simulink model "intelligent_improved_acceleration_function"  (R2024b)
settings: Solver=VariableStepAuto  StartTime=0.0  StopTime=80  RelTol=1e-3
libraries: SignalEditorBlockLib x6
settings Model: Creator=ky  LastModifiedBy=ky

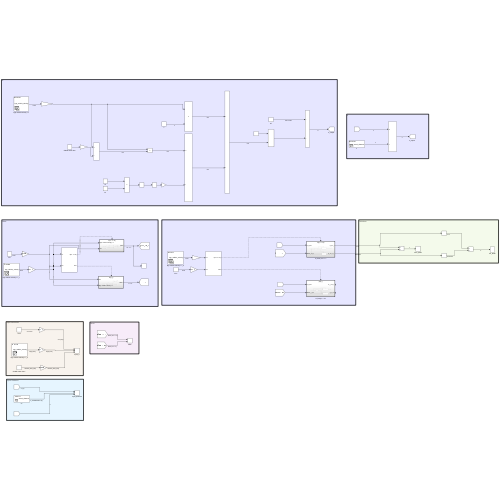
[thumbnail: Simulink's stored preview of the top-level diagram]
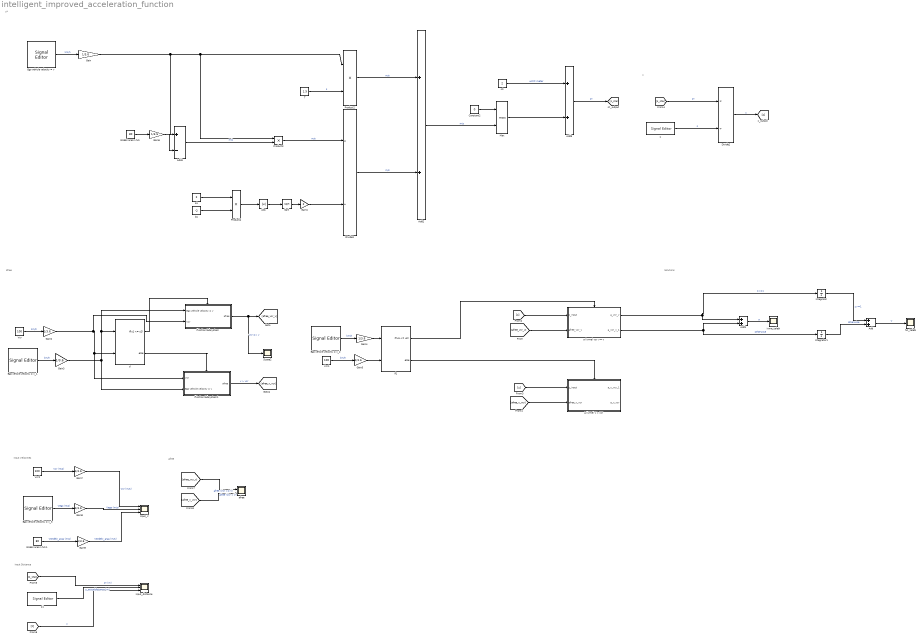
== system intelligent_improved_acceleration_function ==
  note: afree
  note: Solutions
  note: Input Distance
  note: Input Velocities
  note: s*
  note: z
  note: afree
  Abs : Abs  SaturateOnIntegerOverflow=off
  Add{,1..3} (4 alike) : Sum
  Add4 : Sum  Inputs=+-
  Constant2 : Constant  Value=0
  Divide2 : Product  Inputs=*/
  Divide3 : Product  Inputs=*/
  Ego vehicle velocity = v : SignalEditorBlockLib/Signal Editor  FileName=C:\Users\ky\Desktop\MATLAB\otonom_surus\ego_vehicle_velocity.mat  ActiveScenario=Scenario  ActiveSignal=ego_vehicle_velocity  IsBus=off  OutputBusObjectStr=Bus: BusObject  SampleTime=0  ZeroCross=off  OutputAfterFinalValue=Setting to zero  Unit=km/h  PreserveSignalName=on  ApplySigPropsToAllScenarios=on  ApplySigPropsToAllSignals=off
  Ego vehicle velocity = v_1 : SignalEditorBlockLib/Signal Editor  FileName=C:\Users\ky\Desktop\MATLAB\otonom_surus\ego_vehicle_velocity.mat  ActiveScenario=Scenario  ActiveSignal=ego_vehicle_velocity  IsBus=off  OutputBusObjectStr=Bus: BusObject  SampleTime=0  ZeroCross=off  OutputAfterFinalValue=Setting to zero  Unit=km/h  PreserveSignalName=on  ApplySigPropsToAllScenarios=on  ApplySigPropsToAllSignals=off
  Ego vehicle velocity = v_2 : SignalEditorBlockLib/Signal Editor  FileName=C:\Users\ky\Desktop\MATLAB\otonom_surus\ego_vehicle_velocity.mat  ActiveScenario=Scenario  ActiveSignal=ego_vehicle_velocity  IsBus=off  OutputBusObjectStr=Bus: BusObject  SampleTime=0  ZeroCross=off  OutputAfterFinalValue=Setting to zero  Unit=km/h  PreserveSignalName=on  ApplySigPropsToAllScenarios=on  ApplySigPropsToAllSignals=off
  Ego vehicle velocity = v_3 : SignalEditorBlockLib/Signal Editor  FileName=C:\Users\ky\Desktop\MATLAB\otonom_surus\ego_vehicle_velocity.mat  ActiveScenario=Scenario  ActiveSignal=ego_vehicle_velocity  IsBus=off  OutputBusObjectStr=Bus: BusObject  SampleTime=0  ZeroCross=off  OutputAfterFinalValue=Setting to zero  Unit=km/h  PreserveSignalName=on  ApplySigPropsToAllScenarios=on  ApplySigPropsToAllSignals=off
  Gain{,2..9} (9 alike) : Gain  Gain=1/3.6
  Gain1 : Gain  Gain=2
  If : If  NumInputs=2  IfExpression=u1 <= u2
  If Action Subsystem : Subsystem  TreatAsAtomicUnit=on
  If Action Subsystem1 : Subsystem  TreatAsAtomicUnit=on
  If1 : If  NumInputs=2  IfExpression=u1 <= u2
  Input_V : Scope  NumInputPorts=3
  Input_distance : Scope  NumInputPorts=3
  Integrator : Integrator
  Integrator1 : Integrator
  Max : MinMax  Function=max  Inputs=2
  Product2 : Product
  Product3 : Product
  Product4 : Product
  Scope2 : Scope
  Sqrt : Sqrt
  T : Constant  Value=1.5
  Vcr : Constant  Value=100
  Vcr1 : Constant  Value=100
  Vcr2 : Constant  Value=100
  a (ivme) v > vcr : Subsystem  TreatAsAtomicUnit=on
  a (ivme) vcr >= v : Subsystem  TreatAsAtomicUnit=on
  a1 : Constant  Value=2
  afree : Scope  NumInputPorts=2
  b1 : Constant  Value=-2
  hız_talebi : Scope
  ivme_talebi : Scope
  s : SignalEditorBlockLib/Signal Editor  FileName=C:\Users\ky\Desktop\MATLAB\otonom_surus\actual_distance.mat  ActiveScenario=Scenario  ActiveSignal=actual_distance  IsBus=off  OutputBusObjectStr=Bus: BusObject  SampleTime=0  ZeroCross=off  OutputAfterFinalValue=Setting to zero  Unit=m  PreserveSignalName=on  ApplySigPropsToAllScenarios=on  ApplySigPropsToAllSignals=off
  s0 : Constant  Value=2
  s1 : SignalEditorBlockLib/Signal Editor  FileName=C:\Users\ky\Desktop\MATLAB\otonom_surus\actual_distance.mat  ActiveScenario=Scenario  ActiveSignal=actual_distance  IsBus=off  OutputBusObjectStr=Bus: BusObject  SampleTime=0  ZeroCross=off  OutputAfterFinalValue=Setting to zero  Unit=m  PreserveSignalName=on  ApplySigPropsToAllScenarios=on  ApplySigPropsToAllSignals=off
  öndeki aracın hızı : Constant  Value=80
  öndeki aracın hızı1 : Constant  Value=80
  wires:
  Vcr/1 -> Gain2/1  "km/h"
  s1/1 -> Input_distance/2  "s_actualdistance (m)"
  Add4/1 -> Product3/2  "m/s"
  Divide2/1 -> [z]  "z"
  Product3/1 -> Divide3/1  "m/s"
  öndeki aracın hızı1/1 -> Gain9/1  "Vöndeki_araç (m/s)"
  a (ivme) vcr >= v/2(a_vcr_v_1) -> Add1/2, Integrator1/1  "otherwise"
  Product2/1 -> Add2/1  "m/s"
  Ego vehicle velocity = v_1/1 -> Gain3/1  "km/h"
  öndeki aracın hızı/1 -> Gain6/1
  Gain3/1 -> If Action Subsystem1/2(Ego vehicle velocity = v), If Action Subsystem/1(Ego vehicle velocity = v), If/1
  Gain8/1 -> Input_V/2  "Vego (m/s)"
  Add3/1 -> [s_star]  "s*"
  Vcr2/1 -> Gain7/1  "Vcr (m/s)"
  Gain5/1 -> If1/2
  If Action Subsystem1/1(afree) -> [afree_v_vcr]  "v > vcr"
  Abs/1 -> Sqrt/1
  If Action Subsystem/1(afree) -> Scope2/1, [afree_vcr_v]  "vcr => v"
  a (ivme) vcr >= v/1(a_vcr_v) -> Integrator/1, Add1/1  "z>=1"
  Gain4/1 -> If1/1
  [afree_v_vcr] -> a (ivme) v > vcr/2(afree_v_vcr)
  b1/1 -> Product4/2
  Ego vehicle velocity = v_3/1 -> Gain8/1  "Vego (m/s)"
  T/1 -> Product2/2  "s"
  [s_star] -> Divide2/1  "s*"
  Gain/1 -> Add4/1, Product2/1, Product3/1
  Divide3/1 -> Add2/2  "m/s"
  Add2/1 -> Max/2  "m/s"
  s0/1 -> Add3/1  "unit= meter"
  [afree_vcr_v] -> a (ivme) vcr >= v/2(afree_vcr_v)
  If/2 -> If Action Subsystem1/Action
  Gain9/1 -> Input_V/3  "Vöndeki_araç (m/s)"
  [z] -> a (ivme) vcr >= v/1(z_input)
  Constant2/1 -> Max/1
  [z] -> a (ivme) v > vcr/1(z_input)
  Ego vehicle velocity = v/1 -> Gain/1  "km/h"
  Gain7/1 -> Input_V/1  "Vcr (m/s)"
  [s_star] -> Input_distance/1  "s* (m)"
  Sqrt/1 -> Gain1/1
  Gain2/1 -> If Action Subsystem/2(Vcr), If Action Subsystem1/1(Vcr), If/2
  Product4/1 -> Abs/1
  Max/1 -> Add3/2
  Ego vehicle velocity = v_2/1 -> Gain4/1  "km/h"
  s/1 -> Divide2/2  "s"
  If1/1 -> a (ivme) vcr >= v/Action
  [z] -> Input_distance/3  "z"
  If1/2 -> a (ivme) v > vcr/Action
  a1/1 -> Product4/1
  Vcr1/1 -> Gain5/1  "km/h"
  Integrator/1 -> Add/1  "z>=1"
  Gain1/1 -> Divide3/2
  Add1/1 -> ivme_talebi/1  "a"
  Gain6/1 -> Add4/2
  If/1 -> If Action Subsystem/Action
  Add/1 -> hız_talebi/1  "V"
  Integrator1/1 -> Add/2  "otherwise"
  [afree_vcr_v] -> afree/1  "afree (Vcr >= V)"
  [afree_v_vcr] -> afree/2  "afree (Vcr < V)"

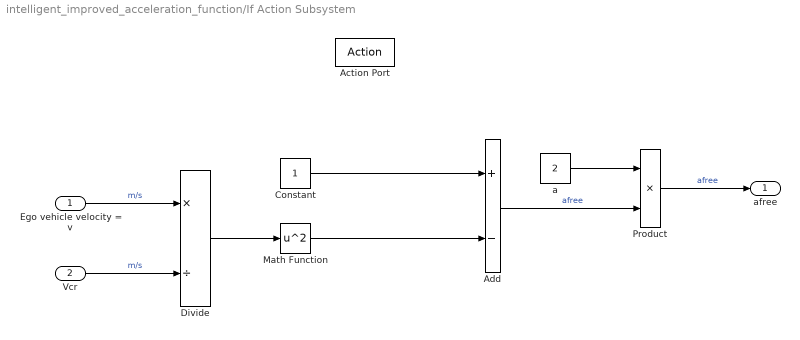
== system intelligent_improved_acceleration_function/If Action Subsystem ==
  Ego vehicle velocity = v : Inport
  Vcr : Inport  Port=2
  Action Port : ActionPort  ActionPortLabel=if(u1 <= u2)
  Add : Sum  Inputs=+-
  Constant : Constant
  Divide : Product  Inputs=*/
  Math Function : Math  Operator=square
  Product : Product
  a : Constant  Value=2
  afree : Outport
  wires:
  Constant/1 -> Add/1
  Math Function/1 -> Add/2
  Divide/1 -> Math Function/1
  a/1 -> Product/1
  Vcr/1 -> Divide/2  "m/s"
  Product/1 -> afree/1  "afree"
  Add/1 -> Product/2  "afree"
  Ego vehicle velocity = v/1 -> Divide/1  "m/s"

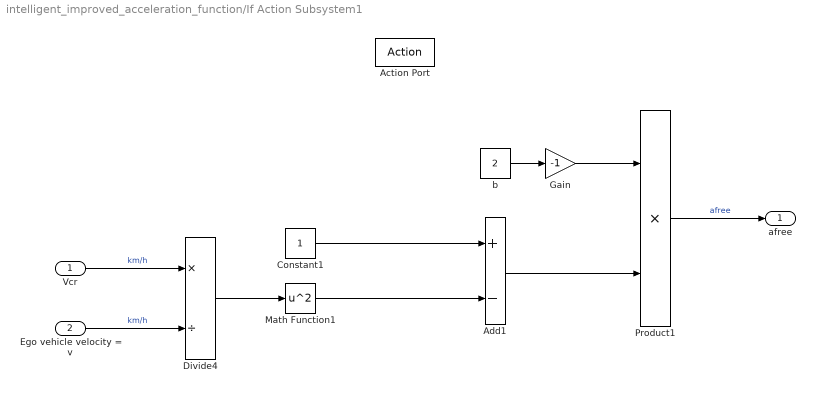
== system intelligent_improved_acceleration_function/If Action Subsystem1 ==
  Vcr : Inport
  Ego vehicle velocity = v : Inport  Port=2
  Action Port : ActionPort  ActionPortLabel=else
  Add1 : Sum  Inputs=+-
  Constant1 : Constant
  Divide4 : Product  Inputs=*/
  Gain : Gain  Gain=-1
  Math Function1 : Math  Operator=square
  Product1 : Product
  b : Constant  Value=2
  afree : Outport
  wires:
  Gain/1 -> Product1/1
  b/1 -> Gain/1
  Vcr/1 -> Divide4/1  "km/h"
  Ego vehicle velocity = v/1 -> Divide4/2  "km/h"
  Product1/1 -> afree/1  "afree"
  Add1/1 -> Product1/2
  Constant1/1 -> Add1/1
  Math Function1/1 -> Add1/2
  Divide4/1 -> Math Function1/1

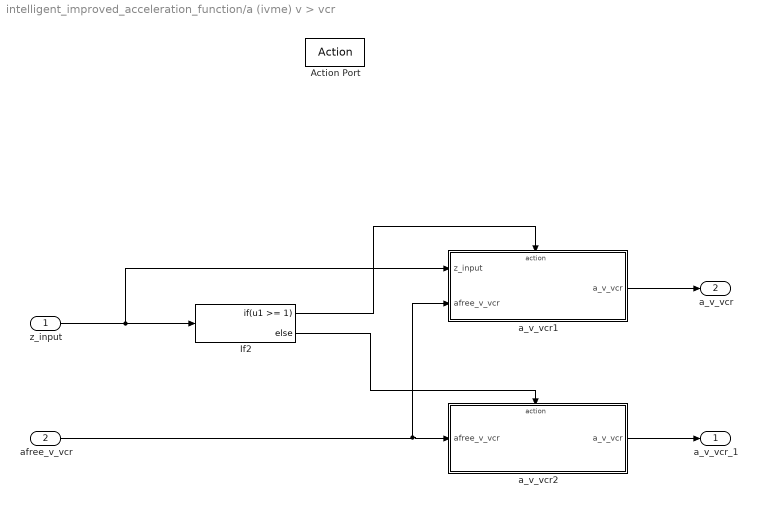
== system intelligent_improved_acceleration_function/a (ivme) v > vcr ==
  z_input : Inport
  afree_v_vcr : Inport  Port=2
  Action Port : ActionPort  ActionPortLabel=else
  If2 : If  IfExpression=u1 >= 1
  a_v_vcr1 : Subsystem  TreatAsAtomicUnit=on
  a_v_vcr2 : Subsystem  TreatAsAtomicUnit=on
  a_v_vcr_1 : Outport
  a_v_vcr : Outport  Port=2
  wires:
  z_input/1 -> a_v_vcr1/1(z_input), If2/1
  If2/1 -> a_v_vcr1/Action
  afree_v_vcr/1 -> a_v_vcr2/1(afree_v_vcr), a_v_vcr1/2(afree_v_vcr)
  If2/2 -> a_v_vcr2/Action
  a_v_vcr1/1(a_v_vcr) -> a_v_vcr/1
  a_v_vcr2/1(a_v_vcr) -> a_v_vcr_1/1

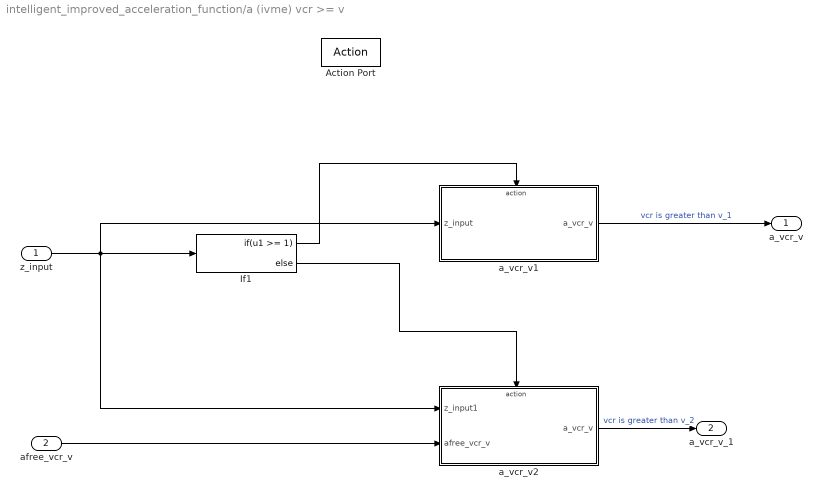
== system intelligent_improved_acceleration_function/a (ivme) vcr >= v ==
  z_input : Inport
  afree_vcr_v : Inport  Port=2
  Action Port : ActionPort  ActionPortLabel=if(u1 <= u2)
  If1 : If  IfExpression=u1 >= 1
  a_vcr_v1 : Subsystem  TreatAsAtomicUnit=on
  a_vcr_v2 : Subsystem  TreatAsAtomicUnit=on
  a_vcr_v : Outport
  a_vcr_v_1 : Outport  Port=2
  wires:
  z_input/1 -> a_vcr_v2/1(z_input1), a_vcr_v1/1(z_input), If1/1
  afree_vcr_v/1 -> a_vcr_v2/2(afree_vcr_v)
  If1/1 -> a_vcr_v1/Action
  If1/2 -> a_vcr_v2/Action
  a_vcr_v1/1(a_vcr_v) -> a_vcr_v/1  "vcr is greater than v_1"
  a_vcr_v2/1(a_vcr_v) -> a_vcr_v_1/1  "vcr is greater than v_2"

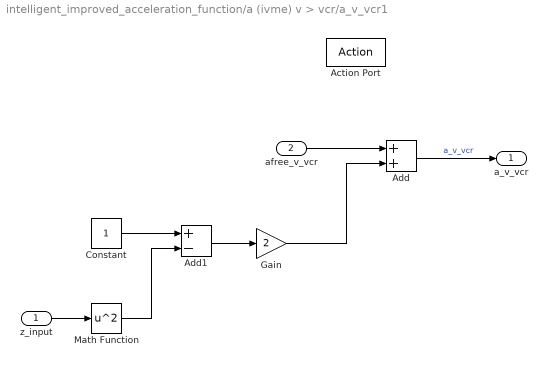
== system intelligent_improved_acceleration_function/a (ivme) v > vcr/a_v_vcr1 ==
  z_input : Inport
  afree_v_vcr : Inport  Port=2
  Action Port : ActionPort  ActionPortLabel=if(u1 >= 1)
  Add : Sum
  Add1 : Sum  Inputs=+-
  Constant : Constant
  Gain : Gain  Gain=2
  Math Function : Math  Operator=square
  a_v_vcr : Outport
  wires:
  Add/1 -> a_v_vcr/1  "a_v_vcr"
  afree_v_vcr/1 -> Add/1
  Add1/1 -> Gain/1
  Gain/1 -> Add/2
  z_input/1 -> Math Function/1
  Math Function/1 -> Add1/2
  Constant/1 -> Add1/1

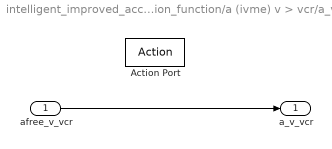
== system intelligent_improved_acceleration_function/a (ivme) v > vcr/a_v_vcr2 ==
  afree_v_vcr : Inport
  Action Port : ActionPort  ActionPortLabel=else
  a_v_vcr : Outport
  wires:
  afree_v_vcr/1 -> a_v_vcr/1

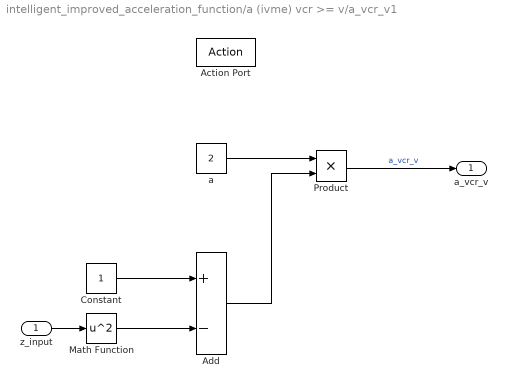
== system intelligent_improved_acceleration_function/a (ivme) vcr >= v/a_vcr_v1 ==
  z_input : Inport
  Action Port : ActionPort  ActionPortLabel=if(u1 >= 1)
  Add : Sum  Inputs=+-
  Constant : Constant
  Math Function : Math  Operator=square
  Product : Product
  a : Constant  Value=2
  a_vcr_v : Outport
  wires:
  Constant/1 -> Add/1
  Add/1 -> Product/2
  Product/1 -> a_vcr_v/1  "a_vcr_v"
  Math Function/1 -> Add/2
  a/1 -> Product/1
  z_input/1 -> Math Function/1

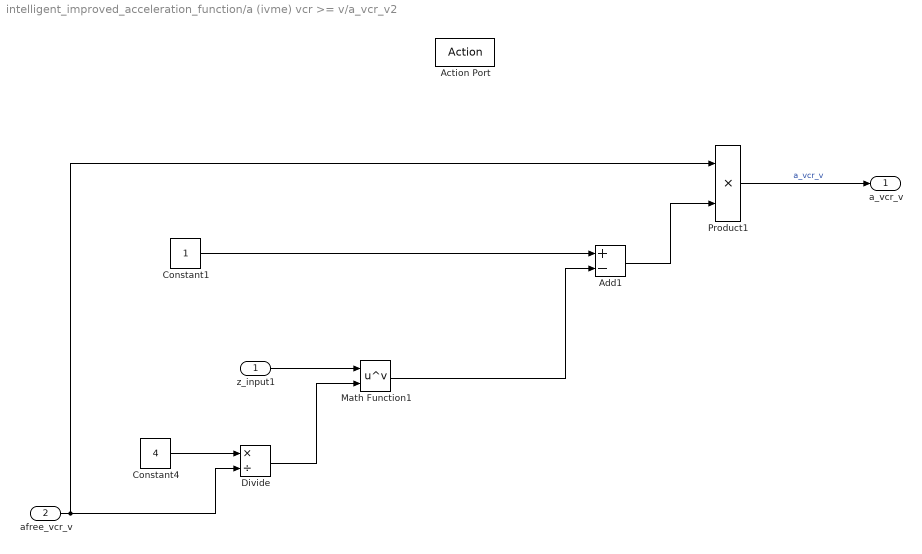
== system intelligent_improved_acceleration_function/a (ivme) vcr >= v/a_vcr_v2 ==
  z_input1 : Inport
  afree_vcr_v : Inport  Port=2
  Action Port : ActionPort  ActionPortLabel=else
  Add1 : Sum  Inputs=+-
  Constant1 : Constant
  Constant4 : Constant  Value=4
  Divide : Product  Inputs=*/
  Math Function1 : Math  Operator=pow
  Product1 : Product
  a_vcr_v : Outport
  wires:
  Divide/1 -> Math Function1/2
  afree_vcr_v/1 -> Product1/1, Divide/2
  Add1/1 -> Product1/2
  Product1/1 -> a_vcr_v/1  "a_vcr_v"
  Math Function1/1 -> Add1/2
  z_input1/1 -> Math Function1/1
  Constant1/1 -> Add1/1
  Constant4/1 -> Divide/1
